simulink model "Simulacija"  (Simulink 8.3)
settings: Solver=ode45  StartTime=0.0  StopTime=0.5  MaxStep=1e-4  RelTol=1e-3
InitFcn:
  | podatki
values from neighbouring files (symbols this model uses):
  Clark = (2/3)*[1 -0.5 -0.5; 0 sqrt(3)/2 -sqrt(3)/2; 0.5 0.5 0.5]    [podatki.m]
  J = 0.019    [parametriAM.m]    (also in podatki.m = 0.01)
  k_r = Lm/Lr    (= 0.956308697428)    [podatki.m]
  k_s = Lm/Ls    (= 0.956308697428)    [podatki.m]
  L_rT = Lr-Lm^2/Ls    (= 0.0209325030625)    [podatki.m]
  L_sT = Ls-Lm^2/Lr    (= 0.0209325030625)    [podatki.m]
  Lm = 0.0493    [parametriAM.m]    (also in podatki.m = 0.2342)
  matrikaM = [0 -1; 1 0]    [podatki.m]
  pp = 3    [parametriAM.m]    (also in podatki.m = 2)
  Rr = 0.689    [parametriAM.m]    (also in podatki.m = 2.2959)
  Rs = 0.594    [parametriAM.m]    (also in podatki.m = 3.7)
  UnRMS = 400    [podatki.m]
  we = 2*pi*fe    (= 314.159265359)    [podatki.m]
settings Model: Creator=Vaje  LastModifiedBy=Mitja1
settings OptimizationCC: ExpressionDepthLimit=2147483647
settings DebuggingCC: FcnCallInpInsideContextMsg=UseLocalSettings

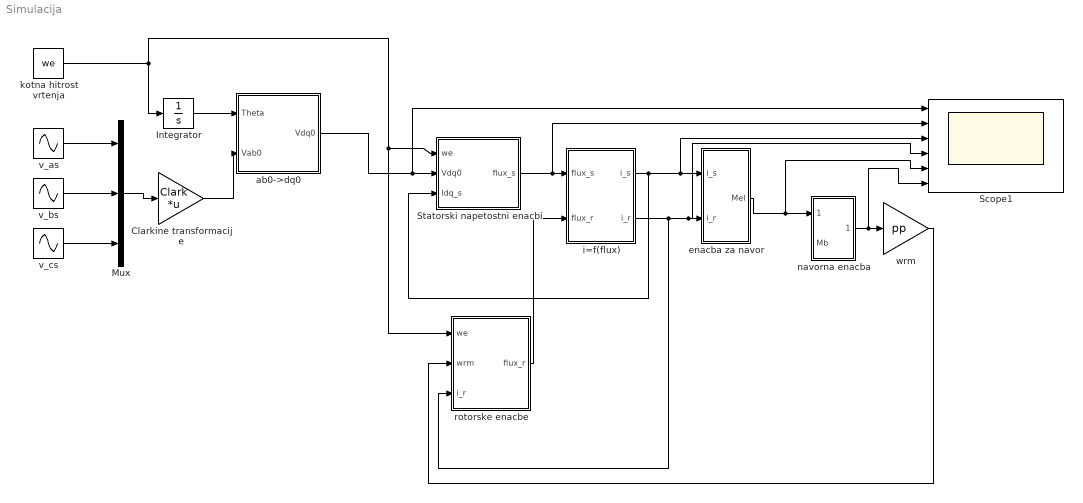
== system Simulacija ==
  Clarkine transformacije : Gain  Gain=Clark  Multiplication=Matrix(K*u)
  Integrator : Integrator
  Mux : Mux  Inputs=3
  Scope1 : Scope  NumInputPorts=6
      settings: YMin=-5~-5~-5~-5~-5~-5  YMax=5~5~5~5~5~5
  Statorski napetostni enacbi : Subsystem
  ab0->dq0 : Subsystem
  enacba za navor : Subsystem
  i=f(flux) : Subsystem
  kotna hitrost vrtenja : Constant  Value=we
  navorna enacba : Subsystem
  rotorske enacbe : Subsystem
  v_as : Sin  Amplitude=UnRMS*sqrt(2/3)  Frequency=we  Phase=pi/2  SampleTime=0
  v_bs : Sin  Amplitude=UnRMS*sqrt(2/3)  Frequency=we  Phase=pi/2 - 2*pi/3  SampleTime=0
  v_cs : Sin  Amplitude=UnRMS*sqrt(2/3)  Frequency=we  Phase=pi/2 +2*pi/3  SampleTime=0
  wrm : Gain  Gain=pp
  wires:
  v_as/1 -> Mux/1
  v_bs/1 -> Mux/2
  v_cs/1 -> Mux/3
  Mux/1 -> Clarkine transformacije/1
  Clarkine transformacije/1 -> ab0->dq0/2(Vab0)
  ab0->dq0/1(Vdq0) -> Scope1/1, Statorski napetostni enacbi/2(Vdq0)
  Integrator/1 -> ab0->dq0/1(Theta)
  Statorski napetostni enacbi/1(flux_s) -> Scope1/2, i=f(flux)/1(flux_s)
  i=f(flux)/1(i_s) -> Statorski napetostni enacbi/3(Idq_s), Scope1/3, enacba za navor/1(i_s)
  i=f(flux)/2(i_r) -> Scope1/4, enacba za navor/2(i_r), rotorske enacbe/3(i_r)
  enacba za navor/1(Mel) -> Scope1/5, navorna enacba/1(Mel)
  navorna enacba/1(wrm) -> Scope1/6, wrm/1
  kotna hitrost vrtenja/1 -> Integrator/1, rotorske enacbe/1(we), Statorski napetostni enacbi/1(we)
  wrm/1 -> rotorske enacbe/2(wrm)
  rotorske enacbe/1(flux_r) -> i=f(flux)/2(flux_r)

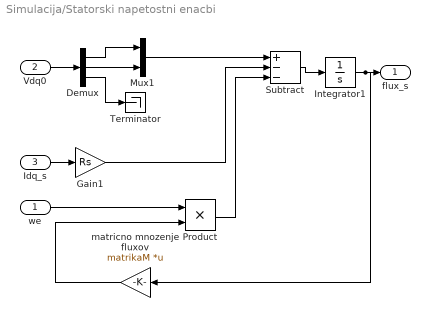
== system Simulacija/Statorski napetostni enacbi ==
  we : Inport
  Vdq0 : Inport  Port=2
  Idq_s : Inport  Port=3
  Demux : Demux  Outputs=3
  Gain1 : Gain  Gain=Rs
  Integrator1 : Integrator
  Mux1 : Mux  Inputs=2
  Product : Product  RndMeth=Zero
  Subtract : Sum  Inputs=+--
  Terminator : Terminator
  matricno mnozenje fluxov : Gain  Gain=matrikaM  Multiplication=Matrix(K*u)
  flux_s : Outport
  wires:
  Demux/3 -> Terminator/1
  Demux/1 -> Mux1/1
  Demux/2 -> Mux1/2
  Mux1/1 -> Subtract/1
  Subtract/1 -> Integrator1/1
  matricno mnozenje fluxov/1 -> Product/2
  we/1 -> Product/1
  Vdq0/1 -> Demux/1
  Integrator1/1 -> flux_s/1, matricno mnozenje fluxov/1
  Idq_s/1 -> Gain1/1
  Product/1 -> Subtract/3
  Gain1/1 -> Subtract/2

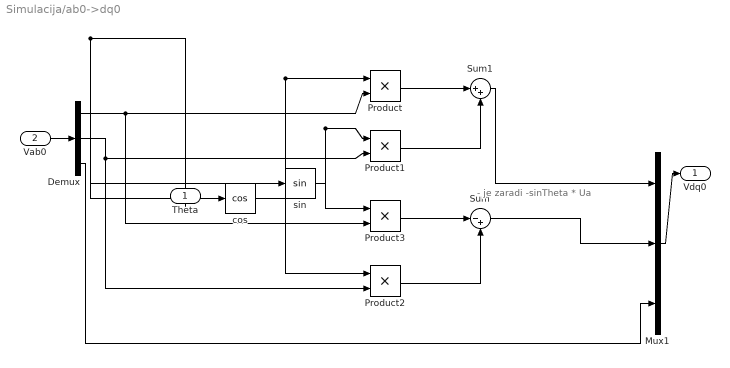
== system Simulacija/ab0->dq0 ==
  note: - je zaradi -sinTheta * Ua
  Theta : Inport
  Vab0 : Inport  Port=2
  Demux : Demux  Outputs=3
  Mux1 : Mux  Inputs=3
  Product{,1..3} (4 alike) : Product  RndMeth=Zero
  Sum : Sum  Inputs=|-+
  Sum1 : Sum  Inputs=|++
  cos : Trigonometry  Operator=cos
  sin : Trigonometry
  Vdq0 : Outport
  wires:
  Theta/1 -> cos/1, sin/1
  Demux/3 -> Mux1/3
  Sum/1 -> Mux1/2
  Vab0/1 -> Demux/1
  Sum1/1 -> Mux1/1
  Mux1/1 -> Vdq0/1
  Demux/1 -> Product/2, Product3/2
  cos/1 -> Product/1, Product2/1
  Demux/2 -> Product2/2, Product1/2
  Product1/1 -> Sum1/2
  Product/1 -> Sum1/1
  sin/1 -> Product3/1, Product1/1
  Product2/1 -> Sum/2
  Product3/1 -> Sum/1

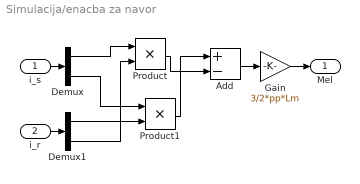
== system Simulacija/enacba za navor ==
  i_s : Inport
  i_r : Inport  Port=2
  Add : Sum  Inputs=+-
  Demux : Demux  Outputs=2
  Demux1 : Demux  Outputs=2
  Gain : Gain  Gain=3/2*pp*Lm
  Product : Product  RndMeth=Zero
  Product1 : Product  RndMeth=Zero
  Mel : Outport
  wires:
  i_s/1 -> Demux/1
  i_r/1 -> Demux1/1
  Gain/1 -> Mel/1
  Add/1 -> Gain/1
  Product1/1 -> Add/1
  Demux/1 -> Product/1
  Demux1/2 -> Product/2
  Demux1/1 -> Product1/2
  Demux/2 -> Product1/1
  Product/1 -> Add/2

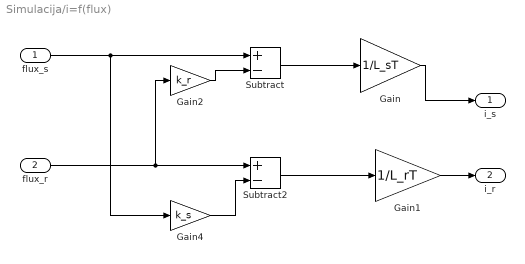
== system Simulacija/i=f(flux) ==
  flux_s : Inport
  flux_r : Inport  Port=2
  Gain : Gain  Gain=1/L_sT
  Gain1 : Gain  Gain=1/L_rT
  Gain2 : Gain  Gain=k_r
  Gain4 : Gain  Gain=k_s
  Subtract : Sum  Inputs=+-
  Subtract2 : Sum  Inputs=+-
  i_s : Outport
  i_r : Outport  Port=2
  wires:
  Subtract/1 -> Gain/1
  Gain4/1 -> Subtract2/2
  flux_s/1 -> Subtract/1, Gain4/1
  Gain/1 -> i_s/1
  flux_r/1 -> Gain2/1, Subtract2/1
  Gain1/1 -> i_r/1
  Gain2/1 -> Subtract/2
  Subtract2/1 -> Gain1/1

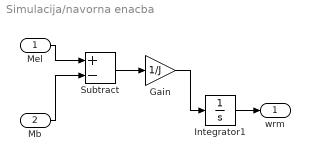
== system Simulacija/navorna enacba ==
  Mel : Inport
  Mb : Inport  Port=2
  Gain : Gain  Gain=1/J
  Integrator1 : Integrator
  Subtract : Sum  Inputs=+-
  wrm : Outport
  wires:
  Mel/1 -> Subtract/1
  Subtract/1 -> Gain/1
  Mb/1 -> Subtract/2
  Integrator1/1 -> wrm/1
  Gain/1 -> Integrator1/1

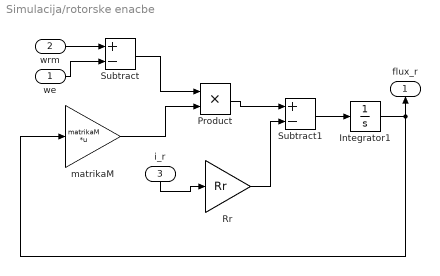
== system Simulacija/rotorske enacbe ==
  we : Inport
  wrm : Inport  Port=2
  i_r : Inport  Port=3
  Integrator1 : Integrator
  Product : Product  RndMeth=Zero
  Rr : Gain  Gain=Rr
  Subtract : Sum  Inputs=+-
  Subtract1 : Sum  Inputs=+-
  matrikaM : Gain  Gain=matrikaM  Multiplication=Matrix(K*u)
  flux_r : Outport
  wires:
  Subtract/1 -> Product/1
  matrikaM/1 -> Product/2
  Product/1 -> Subtract1/1
  Rr/1 -> Subtract1/2
  Subtract1/1 -> Integrator1/1
  Integrator1/1 -> matrikaM/1, flux_r/1
  we/1 -> Subtract/2
  i_r/1 -> Rr/1
  wrm/1 -> Subtract/1
